simulink model "Mounna_DebitMoteur"  (R2025a)
settings: Solver=FixedStepDiscrete  StartTime=0.0  StopTime=SimuPumpStop  FixedStep=0.1  RelTol=1e-6  EnableMultiTasking=on
undefined symbols (not defined in the file): nv_remp, Pamb, PcolTest, PumpedTest, Rair, RegimeTest, Tamb, TempsTest, TimePumpedTest, Vcyl
settings Model: Creator=a030141  LastModifiedBy=Admin
settings SolverCC: AlgebraicLoopSolver=TrustRegion
settings DataIOCC: LimitDataPoints=on  SaveFormat=Array  SignalLoggingSaveFormat=ModelDataLogs  ReturnWorkspaceOutputs=off  SignalLoggingName=sigsOut
settings OptimizationCC: InitFltsAndDblsToZero=on  LifeSpan=inf
settings DebuggingCC: SaveWithParameterizedLinksMsg=none  UnderspecifiedInitializationDetection=Classic  MergeDetectMultiDrivingBlocksExec=none  SignalResolutionControl=TryResolveAllWithWarning  MultiTaskDSMMsg=warning  MultiTaskCondExecSysMsg=none  FcnCallInpInsideContextMsg=warning  UnconnectedInputMsg=warning  UnconnectedOutputMsg=warning  UnconnectedLineMsg=warning  SFUnexpectedBacktrackingDiag=warning  SFNoUnconditionalDefaultTransitionDiag=warning  SFExecutionAtInitializationDiag=none  ArithmeticOperatorsInVariantConditions=warning
settings HardwareCC: ProdBitPerPointer=32.0  ProdBitPerSizeT=32.0  ProdBitPerPtrDiffT=32.0  ProdLargestAtomicFloat=None  ProdIntDivRoundTo=Undefined  ProdEndianess=Unspecified  ProdWordSize=32.0  ProdHWDeviceType=32-bit Generic  TargetUnknown=on
settings ModelReferenceCC: PropagateSignalLabelsOutOfModel=off
settings RTWCC: GPUComputeCapability=3.5
settings CodeAppCC: StateflowObjectComments=on
settings GRTTargetCC: TargetFcnLib=ansi_tfl_tmw.mat  TargetLangStandard=C89/C90 (ANSI)  CombineOutputUpdateFcns=off  GRTInterface=on
settings ConfigComp: CovMetricSettings=dw  CovSaveCumulativeToWorkspaceVar=on  CovSaveSingleToWorkspaceVar=on

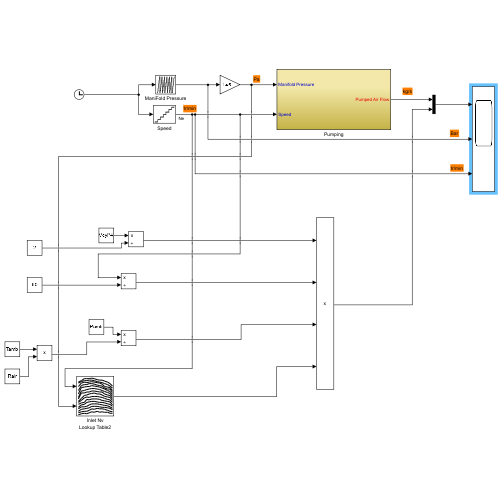
[thumbnail: Simulink's stored preview of the top-level diagram]
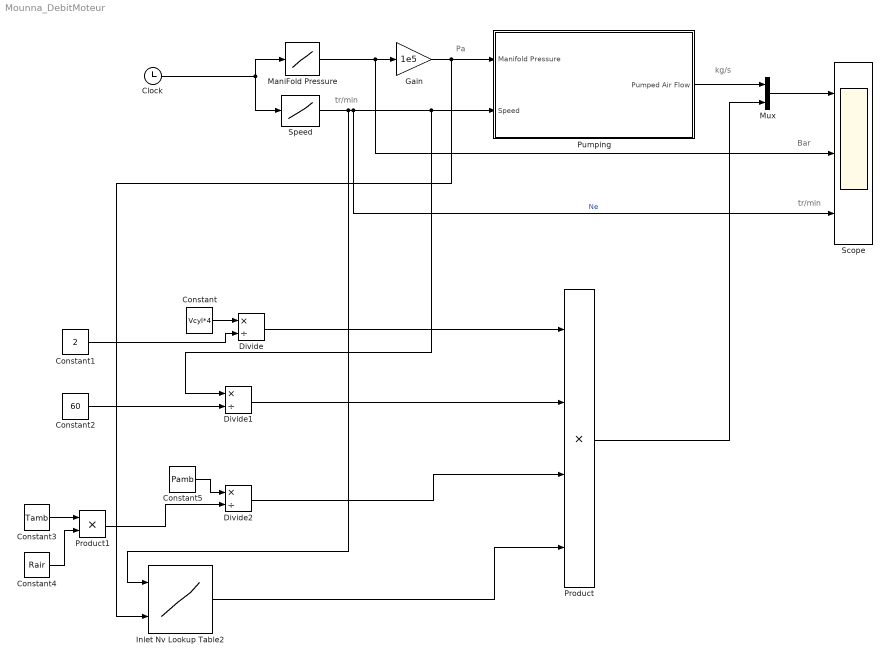
== system Mounna_DebitMoteur ==
  note: kg/s
  note: Pa
  note: Bar
  note: tr/min
  note: tr/min
  Clock : Clock
  Constant : Constant  Value=Vcyl*4
  Constant1 : Constant  Value=2
  Constant2 : Constant  Value=60
  Constant3 : Constant  Value=Tamb
  Constant4 : Constant  Value=Rair
  Constant5 : Constant  Value=Pamb
  Divide : Product  Inputs=*/
  Divide1 : Product  Inputs=*/
  Divide2 : Product  Inputs=*/
  Gain : Gain  Gain=1e5  SaturateOnIntegerOverflow=on  OutDataTypeStr=Inherit: Same as input  ParamDataTypeStr=Inherit: Same as input
  Inlet Nv Lookup Table2 : Lookup2D  RowIndex=Ne_remp  ColumnIndex=Pcol_remp  Table=nv_remp
  ManiFold Pressure : Lookup  InputValues=TempsTest  Table=PcolTest
  Mux : Mux  Inputs=2
  Product : Product  Inputs=4
  Product1 : Product
  Pumping : Subsystem
  Scope : Scope  NumInputPorts=3
      settings: TimeSpan=596.5  Title=Debit [kg/s]  ActiveDisplayYMinimum=-0.0052707656250000007  ActiveDisplayYMaximum=0.05977819550304881
  Speed : Lookup  InputValues=TempsTest  Table=RegimeTest
  wires:
  Speed/1 -> Inlet Nv Lookup Table2/1, Scope/3, Divide1/1, Pumping/2(Speed)  "Ne"
  Clock/1 -> ManiFold Pressure/1, Speed/1
  ManiFold Pressure/1 -> Gain/1, Scope/2
  Mux/1 -> Scope/1
  Pumping/1(Pumped Air Flow) -> Mux/1
  Constant/1 -> Divide/1
  Constant1/1 -> Divide/2
  Divide/1 -> Product/1
  Constant2/1 -> Divide1/2
  Divide1/1 -> Product/2
  Constant3/1 -> Product1/1
  Constant4/1 -> Product1/2
  Product1/1 -> Divide2/2
  Divide2/1 -> Product/3
  Inlet Nv Lookup Table2/1 -> Product/4
  Product/1 -> Mux/2
  Gain/1 -> Inlet Nv Lookup Table2/2, Pumping/1(Manifold Pressure)
  Constant5/1 -> Divide2/1

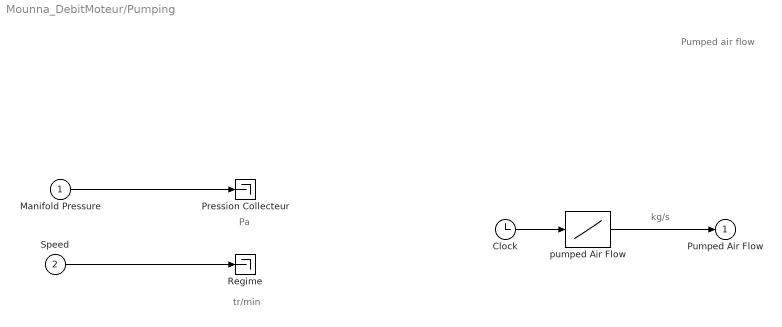
== system Mounna_DebitMoteur/Pumping ==
  note: Pumped air flow
  note: kg/s
  note: Pa
  note: tr/min
  Manifold Pressure : Inport
  Speed : Inport  Port=2
  Clock : Clock
  Pression Collecteur : Terminator
  Regime : Terminator
  pumped Air Flow : Lookup  InputValues=TimePumpedTest  Table=PumpedTest
  Pumped Air Flow : Outport
  wires:
  Manifold Pressure/1 -> Pression Collecteur/1
  Speed/1 -> Regime/1
  pumped Air Flow/1 -> Pumped Air Flow/1
  Clock/1 -> pumped Air Flow/1
